simulink model "Consensus_Swarm"  (R2023b)
settings: Solver=ode3  StartTime=0.0  StopTime=inf  FixedStep=0.001  RelTol=1e-3
values from neighbouring files (symbols this model uses):
  g = 9.8    [Parameters.m]
  Ic = [2 0 0; 0 2 0; 0 0 4]    [Parameters.m]
  m = 1    [Parameters.m]
  M_RB = [eye(3), zeros(3); zeros(3), I]    [Parameters.m]
  SAVE_SPACE = 5    [Parameters.m]
  STEP_SIZE = 1    [Parameters.m]
libraries: simulink_extras x36, slpidlib x36, aerolibutil x12, vrlib x7
(part 1 of 6)
settings Model: Creator=angel  LastModifiedBy=angel

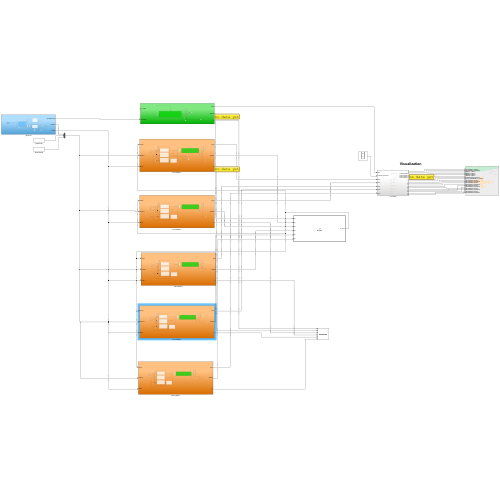
[thumbnail: Simulink's stored preview of the top-level diagram]
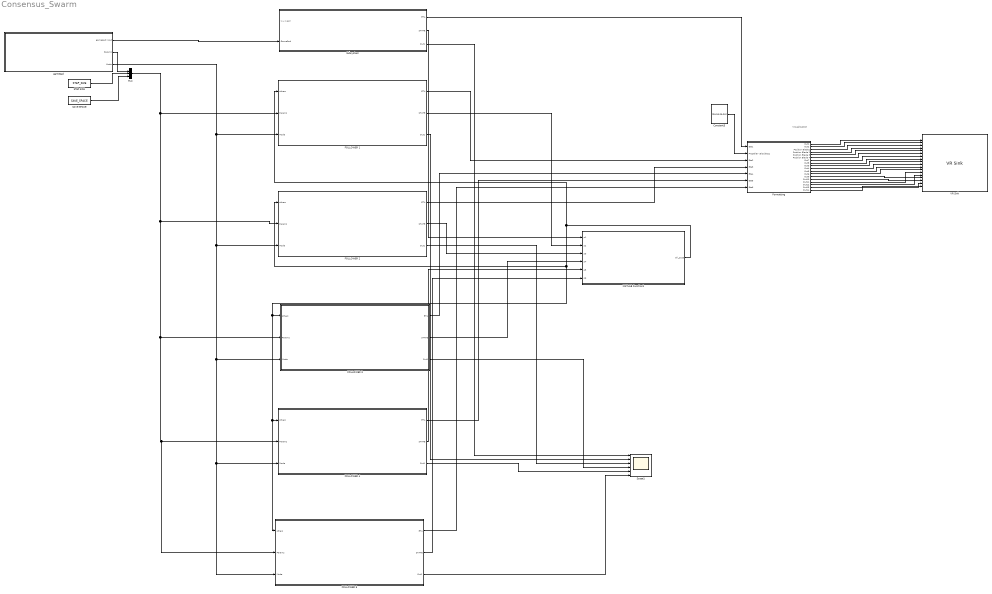
== system Consensus_Swarm ==
  note: Visualization
  Constant3 : Constant  Value=[20;20;20;20]  VectorParams1D=off
  FOLLOWER 1 : Subsystem
  FOLLOWER 2 : Subsystem
  FOLLOWER 3 : Subsystem
  FOLLOWER 4 : Subsystem
  FOLLOWER 5 : Subsystem
  Formatting : Subsystem
  MATLAB Function1 : MATLAB Function  TreatAsAtomicUnit=on
  Mux : Mux  Inputs=3
  SAVE SPACE : Constant  Value=SAVE_SPACE
  STEP SIZE : Constant  Value=STEP_SIZE
  Scope1 : Scope  NumInputPorts=6
  Subsystem : Subsystem
  VR Sink : vrlib/VR Sink  InstantiateOnLoad=on  SampleTime=12*0.005  ViewEnable=on  RemoteChange=off  RemoteView=off  FieldsWritten=QuadBody1.rotation.4.1.1.double#QuadBody1.translation.3.1.1.double#Blade1.rotation.4.1.1.double#Blade3.rotation.4.1.1.double#Blade2.rotation.4.1.1.double#Blade4.rotation.4.1.1.double#IsoNoRotation.position.3.1.1.double#OnQuadNoRotation.position.3.1.1.double#QuadBody2.rotation.4.1.1.double#QuadBody2.translation.3.1.1.double#QuadBody3.rotation.4.1.1.double#QuadBody3.translation.3.1.1.double#QuadBody5.rotation.4.1.1.double#QuadBody5.translation.3.1.1.double#QuadBody4.rotation.4.1.1.double#QuadBody4.translation.3.1.1.double#QuadBody6.rotation.4.1.1.double#QuadBody6.translation.3.1.1.double  WorldFileName=Quadcoptertwo_VR.wrl  AutoView=on  VideoDimensions=[]  AllowVariableSize=off  FigureProperties="{'Position', 'Name', 'Viewpoint', 'CameraBound', 'CameraDirection', 'CameraPosition', 'CameraUpVector', 'ZoomFactor', 'Antialiasing', 'Headlight', 'Lighting', 'NavPanel', 'Sound', 'StatusBar', 'Stereo3D', 'Stereo3DCameraOffset', 'Stereo3DHIT', 'ToolBar', 'Textures', 'Transparency', 'Triad', 'Wireframe', 'NavZones', 'NavMode', 'NavSpeed', 'CaptureFileFormat', 'CaptureFileName', 'Record2DCompressMethod', 'Record2DCompressQuality', 'Record2D', 'Record2DFileName', 'Record2DFPS'; [1.0000000000000000e+00   7.4199999999999932e+01   1.5360000000000000e+03   6.9080000000000007e+02], '', 'Isometric', 'on', [0.0000000000000000e+00   0.0000000000000000e+00  -1.0000000000000000e+00], [0.0000000000000000e+00   0.0000000000000000e+00   6.0000000000000000e+00], [0.0000000000000000e+00   1.0000000000000000e+00   0.0000000000000000e+00], [1.0000000000000000e+00], 'on', 'on', 'on', 'halfbar', 'on', 'on', 'off', [1.0000000149011612e-01], [0.0000000000000000e+00], 'on', 'on', 'on', 'none', 'off', 'off', 'fly', 'normal', 'tif', '%f_anim_%n.tif', 'auto', [7.5000000000000000e+01], 'off', '%f_anim_%n.avi', 'auto'}"
  gamepad : Subsystem
  wires:
  Constant3/1 -> Formatting/2(Propeller velocities1)
  gamepad/2(Params) -> Mux/1
  STEP SIZE/1 -> Mux/2
  Mux/1 -> FOLLOWER 2/2(Params), FOLLOWER 4/2(Params), FOLLOWER 5/2(Params), FOLLOWER 3/2(Params), FOLLOWER 1/2(Params)
  FOLLOWER 3/1(ETA) -> Formatting/5(Eta4)
  FOLLOWER 3/2(STATE) -> MATLAB Function1/4(p4)
  SAVE SPACE/1 -> Mux/3
  MATLAB Function1/1(all_pose) -> FOLLOWER 1/1(others), FOLLOWER 2/1(others), FOLLOWER 5/1(others), FOLLOWER 4/1(others), FOLLOWER 3/1(others)
  FOLLOWER 2/2(STATE) -> MATLAB Function1/3(p3)
  FOLLOWER 1/2(STATE) -> MATLAB Function1/2(p2)
  FOLLOWER 2/1(ETA) -> Formatting/4(Eta3)
  FOLLOWER 1/1(ETA) -> Formatting/3(Eta2)
  gamepad/1(gamepad input) -> Subsystem/2(GamePad)
  Subsystem/1(ETA) -> Formatting/1(Eta1)
  Subsystem/2(STATE) -> MATLAB Function1/1(p1)
  gamepad/3(Mode) -> FOLLOWER 5/3(Mode), FOLLOWER 4/3(Mode), FOLLOWER 3/3(Mode), FOLLOWER 2/3(Mode), FOLLOWER 1/3(Mode)
  Formatting/1(Out1) -> VR Sink/1
  Formatting/2(Out2) -> VR Sink/2
  Formatting/3(Position Blade1) -> VR Sink/3
  Formatting/4(Position Blade 2) -> VR Sink/4
  Formatting/5(Position Blade 3) -> VR Sink/5
  Formatting/6(Position Blade 4) -> VR Sink/6
  Formatting/7(Out7) -> VR Sink/7
  Formatting/8(Out8) -> VR Sink/8
  Formatting/9(Out3) -> VR Sink/9
  Formatting/10(Out4) -> VR Sink/10
  Formatting/11(Out5) -> VR Sink/11
  Formatting/12(Out6) -> VR Sink/12
  Formatting/13(Out9) -> VR Sink/15
  Formatting/14(Out10) -> VR Sink/16
  Formatting/15(Out11) -> VR Sink/13
  Formatting/16(Out12) -> VR Sink/14
  Formatting/17(Out13) -> VR Sink/17
  Formatting/18(Out14) -> VR Sink/18
  FOLLOWER 4/1(ETA) -> Formatting/6(Eta5)
  FOLLOWER 4/2(STATE) -> MATLAB Function1/5(p5)
  FOLLOWER 5/1(ETA) -> Formatting/7(Eta6)
  FOLLOWER 5/2(STATE) -> MATLAB Function1/6(p6)
  FOLLOWER 5/3(Out1) -> Scope1/6
  FOLLOWER 4/3(Out1) -> Scope1/5
  FOLLOWER 3/3(Out1) -> Scope1/4
  FOLLOWER 2/3(Out1) -> Scope1/3
  FOLLOWER 1/3(Out1) -> Scope1/2
  Subsystem/3(Out1) -> Scope1/1

== system Consensus_Swarm/FOLLOWER 1 ==
  others : Inport
  Params : Inport  Port=2
  Mode : Inport  Port=3
  Agent Model : Subsystem
  Demux : Demux
  Demux1 : Demux
  Demux3 : Demux  Outputs=6
  ID : Constant  Value=2
  MATLAB Function : MATLAB Function  TreatAsAtomicUnit=on
  MATLAB Function1 : MATLAB Function  TreatAsAtomicUnit=on
  MATLAB Function10 : MATLAB Function  TreatAsAtomicUnit=on
  MATLAB Function11 : MATLAB Function  TreatAsAtomicUnit=on
  Multiport Switch : MultiPortSwitch  SaturateOnIntegerOverflow=off  InputSameDT=off
  Mux4 : Mux
  Scope : Scope  NumInputPorts=2
  ETA : Outport
  STATE : Outport  Port=2
  Out1 : Outport  Port=3
  wires:
  MATLAB Function11/1(ref) -> Multiport Switch/2
  others/1 -> MATLAB Function10/3(others), MATLAB Function1/2(others), MATLAB Function/2(others), MATLAB Function11/2(others)
  Params/1 -> Demux/1
  ID/1 -> MATLAB Function10/1(id), MATLAB Function/1(id), MATLAB Function11/1(id), MATLAB Function1/1(id)
  Demux/1 -> MATLAB Function/4(d), MATLAB Function11/3(d)
  Demux/2 -> MATLAB Function11/4(phi)
  Demux/4 -> MATLAB Function10/4(safe_space)
  Demux/3 -> MATLAB Function11/5(base_speed), MATLAB Function1/3(base_speed), MATLAB Function/3(base_speed)
  Demux3/3 -> Mux4/3
  MATLAB Function1/1(ref) -> MATLAB Function10/2(ref)
  Mode/1 -> Multiport Switch/1
  MATLAB Function10/1(new_ref) -> Multiport Switch/4
  Agent Model/1(Eta) -> ETA/1, Demux3/1
  Multiport Switch/1 -> Agent Model/1((x,y,z,psi))
  Demux3/1 -> Mux4/1
  Demux3/2 -> Mux4/2
  Mux4/1 -> STATE/1
  Demux3/6 -> Out1/1, Mux4/4
  Demux1/4 -> Scope/1
  MATLAB Function/1(ref) -> Demux1/1, Multiport Switch/3
  MATLAB Function/2(angle) -> Scope/2

== system Consensus_Swarm/FOLLOWER 2 ==
  others : Inport
  Params : Inport  Port=2
  Mode : Inport  Port=3
  Agent Model : Subsystem
  Demux : Demux
  Demux3 : Demux  Outputs=6
  ID : Constant  Value=3
  MATLAB Function : MATLAB Function  TreatAsAtomicUnit=on
  MATLAB Function1 : MATLAB Function  TreatAsAtomicUnit=on
  MATLAB Function10 : MATLAB Function  TreatAsAtomicUnit=on
  MATLAB Function11 : MATLAB Function  TreatAsAtomicUnit=on
  Multiport Switch : MultiPortSwitch  SaturateOnIntegerOverflow=off  InputSameDT=off
  Mux4 : Mux
  ETA : Outport
  STATE : Outport  Port=2
  Out1 : Outport  Port=3
  wires:
  MATLAB Function11/1(ref) -> Multiport Switch/2
  others/1 -> MATLAB Function10/3(others), MATLAB Function1/2(others), MATLAB Function/2(others), MATLAB Function11/2(others)
  Params/1 -> Demux/1
  ID/1 -> MATLAB Function10/1(id), MATLAB Function/1(id), MATLAB Function11/1(id), MATLAB Function1/1(id)
  Demux/1 -> MATLAB Function/4(d), MATLAB Function11/3(d)
  Demux/2 -> MATLAB Function11/4(phi)
  Demux/4 -> MATLAB Function10/4(safe_space)
  Demux/3 -> MATLAB Function11/5(base_speed), MATLAB Function1/3(base_speed), MATLAB Function/3(base_speed)
  Demux3/3 -> Mux4/3
  MATLAB Function/1(ref) -> Multiport Switch/3
  MATLAB Function1/1(ref) -> MATLAB Function10/2(ref)
  Mode/1 -> Multiport Switch/1
  MATLAB Function10/1(new_ref) -> Multiport Switch/4
  Agent Model/1(Eta) -> ETA/1, Demux3/1
  Multiport Switch/1 -> Agent Model/1((x,y,z,psi))
  Demux3/1 -> Mux4/1
  Demux3/2 -> Mux4/2
  Mux4/1 -> STATE/1
  Demux3/6 -> Out1/1, Mux4/4

== system Consensus_Swarm/FOLLOWER 3 ==
  others : Inport
  Params : Inport  Port=2
  Mode : Inport  Port=3
  Agent Model : Subsystem
  Demux : Demux
  Demux3 : Demux  Outputs=6
  ID : Constant  Value=4
  MATLAB Function : MATLAB Function  TreatAsAtomicUnit=on
  MATLAB Function1 : MATLAB Function  TreatAsAtomicUnit=on
  MATLAB Function10 : MATLAB Function  TreatAsAtomicUnit=on
  MATLAB Function11 : MATLAB Function  TreatAsAtomicUnit=on
  Multiport Switch : MultiPortSwitch  SaturateOnIntegerOverflow=off  InputSameDT=off
  Mux4 : Mux
  ETA : Outport
  STATE : Outport  Port=2
  Out1 : Outport  Port=3
  wires:
  MATLAB Function11/1(ref) -> Multiport Switch/2
  others/1 -> MATLAB Function10/3(others), MATLAB Function1/2(others), MATLAB Function/2(others), MATLAB Function11/2(others)
  Params/1 -> Demux/1
  ID/1 -> MATLAB Function10/1(id), MATLAB Function/1(id), MATLAB Function11/1(id), MATLAB Function1/1(id)
  Demux/1 -> MATLAB Function/4(d), MATLAB Function11/3(d)
  Demux/2 -> MATLAB Function11/4(phi)
  Demux/4 -> MATLAB Function10/4(safe_space)
  Demux/3 -> MATLAB Function11/5(base_speed), MATLAB Function/3(base_speed), MATLAB Function1/3(base_speed)
  Demux3/3 -> Mux4/3
  MATLAB Function/1(ref) -> Multiport Switch/3
  MATLAB Function1/1(ref) -> MATLAB Function10/2(ref)
  Mode/1 -> Multiport Switch/1
  MATLAB Function10/1(new_ref) -> Multiport Switch/4
  Agent Model/1(Eta) -> ETA/1, Demux3/1
  Multiport Switch/1 -> Agent Model/1((x,y,z,psi))
  Demux3/1 -> Mux4/1
  Demux3/2 -> Mux4/2
  Mux4/1 -> STATE/1
  Demux3/6 -> Mux4/4, Out1/1

== system Consensus_Swarm/FOLLOWER 4 ==
  others : Inport
  Params : Inport  Port=2
  Mode : Inport  Port=3
  Agent Model : Subsystem
  Demux : Demux
  Demux3 : Demux  Outputs=6
  ID : Constant  Value=5
  MATLAB Function : MATLAB Function  TreatAsAtomicUnit=on
  MATLAB Function1 : MATLAB Function  TreatAsAtomicUnit=on
  MATLAB Function10 : MATLAB Function  TreatAsAtomicUnit=on
  MATLAB Function11 : MATLAB Function  TreatAsAtomicUnit=on
  Multiport Switch : MultiPortSwitch  SaturateOnIntegerOverflow=off  InputSameDT=off
  Mux4 : Mux
  ETA : Outport
  STATE : Outport  Port=2
  Out1 : Outport  Port=3
  wires:
  MATLAB Function11/1(ref) -> Multiport Switch/2
  others/1 -> MATLAB Function10/3(others), MATLAB Function1/2(others), MATLAB Function/2(others), MATLAB Function11/2(others)
  Params/1 -> Demux/1
  ID/1 -> MATLAB Function10/1(id), MATLAB Function/1(id), MATLAB Function11/1(id), MATLAB Function1/1(id)
  Demux/1 -> MATLAB Function/4(d), MATLAB Function11/3(d)
  Demux/2 -> MATLAB Function11/4(phi)
  Demux/4 -> MATLAB Function10/4(safe_space)
  Demux/3 -> MATLAB Function11/5(base_speed), MATLAB Function/3(base_speed), MATLAB Function1/3(base_speed)
  Demux3/3 -> Mux4/3
  MATLAB Function/1(ref) -> Multiport Switch/3
  MATLAB Function1/1(ref) -> MATLAB Function10/2(ref)
  Mode/1 -> Multiport Switch/1
  MATLAB Function10/1(new_ref) -> Multiport Switch/4
  Agent Model/1(Eta) -> ETA/1, Demux3/1
  Multiport Switch/1 -> Agent Model/1((x,y,z,psi))
  Demux3/1 -> Mux4/1
  Demux3/2 -> Mux4/2
  Mux4/1 -> STATE/1
  Demux3/6 -> Out1/1, Mux4/4

== system Consensus_Swarm/FOLLOWER 5 ==
  others : Inport
  Params : Inport  Port=2
  Mode : Inport  Port=3
  Agent Model : Subsystem
  Demux : Demux
  Demux3 : Demux  Outputs=6
  ID : Constant  Value=6
  MATLAB Function : MATLAB Function  TreatAsAtomicUnit=on
  MATLAB Function1 : MATLAB Function  TreatAsAtomicUnit=on
  MATLAB Function10 : MATLAB Function  TreatAsAtomicUnit=on
  MATLAB Function11 : MATLAB Function  TreatAsAtomicUnit=on
  Multiport Switch : MultiPortSwitch  SaturateOnIntegerOverflow=off  InputSameDT=off
  Mux4 : Mux
  ETA : Outport
  STATE : Outport  Port=2
  Out1 : Outport  Port=3
  wires:
  MATLAB Function11/1(ref) -> Multiport Switch/2
  others/1 -> MATLAB Function10/3(others), MATLAB Function1/2(others), MATLAB Function/2(others), MATLAB Function11/2(others)
  Params/1 -> Demux/1
  ID/1 -> MATLAB Function10/1(id), MATLAB Function/1(id), MATLAB Function11/1(id), MATLAB Function1/1(id)
  Demux/1 -> MATLAB Function/4(d), MATLAB Function11/3(d)
  Demux/2 -> MATLAB Function11/4(phi)
  Demux/4 -> MATLAB Function10/4(safe_space)
  Demux/3 -> MATLAB Function11/5(base_speed), MATLAB Function/3(base_speed), MATLAB Function1/3(base_speed)
  Demux3/3 -> Mux4/3
  MATLAB Function/1(ref) -> Multiport Switch/3
  MATLAB Function1/1(ref) -> MATLAB Function10/2(ref)
  Mode/1 -> Multiport Switch/1
  MATLAB Function10/1(new_ref) -> Multiport Switch/4
  Agent Model/1(Eta) -> ETA/1, Demux3/1
  Multiport Switch/1 -> Agent Model/1((x,y,z,psi))
  Demux3/1 -> Mux4/1
  Demux3/2 -> Mux4/2
  Mux4/1 -> STATE/1
  Demux3/6 -> Out1/1, Mux4/4

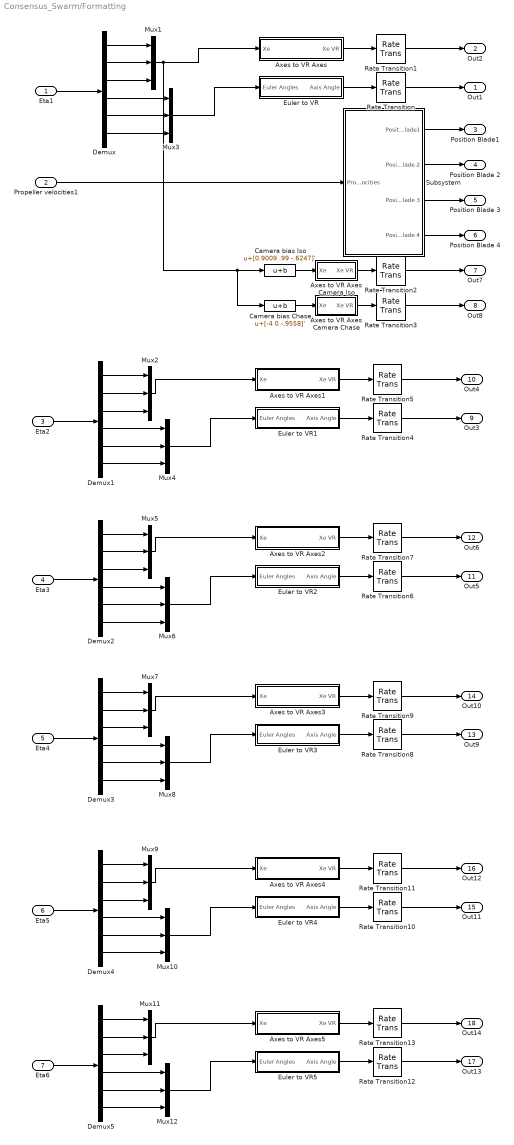
== system Consensus_Swarm/Formatting ==
  Eta1 : Inport
  Propeller velocities1 : Inport  Port=2
  Eta2 : Inport  Port=3
  Eta3 : Inport  Port=4
  Eta4 : Inport  Port=5
  Eta5 : Inport  Port=6
  Eta6 : Inport  Port=7
  Axes to VR Axes : Subsystem
  Axes to VR Axes Camera Chase : Subsystem
  Axes to VR Axes Camera Iso : Subsystem
  Axes to VR Axes1 : Subsystem
  Axes to VR Axes2 : Subsystem
  Axes to VR Axes3 : Subsystem
  Axes to VR Axes4 : Subsystem
  Axes to VR Axes5 : Subsystem
  Camera bias Chase : Bias  Bias=[-4 0 -.9558]'  SaturateOnIntegerOverflow=off
  Camera bias Iso : Bias  Bias=[0.9009 .99 -.6247]'  SaturateOnIntegerOverflow=off
  Demux{,1..5} (6 alike) : Demux  Outputs=6
  Euler to VR : Subsystem
  Euler to VR1 : Subsystem
  Euler to VR2 : Subsystem
  Euler to VR3 : Subsystem
  Euler to VR4 : Subsystem
  Euler to VR5 : Subsystem
  Mux{1..12} (12 alike) : Mux  Inputs=3
  Rate Transition{,1..13} (14 alike) : RateTransition
  Subsystem : Subsystem
  Out1 : Outport
  Out2 : Outport  Port=2
  Position Blade1 : Outport  Port=3
  Position Blade 2 : Outport  Port=4
  Position Blade 3 : Outport  Port=5
  Position Blade 4 : Outport  Port=6
  Out7 : Outport  Port=7
  Out8 : Outport  Port=8
  Out3 : Outport  Port=9
  Out4 : Outport  Port=10
  Out5 : Outport  Port=11
  Out6 : Outport  Port=12
  Out9 : Outport  Port=13
  Out10 : Outport  Port=14
  Out11 : Outport  Port=15
  Out12 : Outport  Port=16
  Out13 : Outport  Port=17
  Out14 : Outport  Port=18
  wires:
  Rate Transition2/1 -> Out7/1
  Propeller velocities1/1 -> Subsystem/1(Propeller velocities)
  Subsystem/3(Position Blade 3) -> Position Blade 3/1
  Subsystem/1(Position Blade1) -> Position Blade1/1
  Mux3/1 -> Euler to VR/1(Euler Angles)
  Camera bias Chase/1 -> Axes to VR Axes Camera Chase/1(Xe)
  Axes to VR Axes Camera Chase/1(Xe VR) -> Rate Transition3/1
  Subsystem/2(Position Blade 2) -> Position Blade 2/1
  Axes to VR Axes Camera Iso/1(Xe VR) -> Rate Transition2/1
  Euler to VR/1(Axis Angle) -> Rate Transition/1
  Axes to VR Axes/1(Xe VR) -> Rate Transition1/1
  Rate Transition1/1 -> Out2/1
  Camera bias Iso/1 -> Axes to VR Axes Camera Iso/1(Xe)
  Mux1/1 -> Camera bias Chase/1, Camera bias Iso/1, Axes to VR Axes/1(Xe)
  Rate Transition3/1 -> Out8/1
  Rate Transition/1 -> Out1/1
  Subsystem/4(Position Blade 4) -> Position Blade 4/1
  Demux/2 -> Mux1/2
  Demux/5 -> Mux3/2
  Demux/3 -> Mux1/3
  Eta1/1 -> Demux/1
  Demux/1 -> Mux1/1
  Demux/4 -> Mux3/1
  Demux/6 -> Mux3/3
  Demux1/3 -> Mux2/3
  Demux1/1 -> Mux2/1
  Euler to VR1/1(Axis Angle) -> Rate Transition4/1
  Mux2/1 -> Axes to VR Axes1/1(Xe)
  Eta2/1 -> Demux1/1
  Axes to VR Axes1/1(Xe VR) -> Rate Transition5/1
  Rate Transition5/1 -> Out4/1
  Mux4/1 -> Euler to VR1/1(Euler Angles)
  Demux1/4 -> Mux4/1
  Demux1/2 -> Mux2/2
  Rate Transition4/1 -> Out3/1
  Demux1/5 -> Mux4/2
  Demux1/6 -> Mux4/3
  Mux6/1 -> Euler to VR2/1(Euler Angles)
  Demux2/6 -> Mux6/3
  Demux2/5 -> Mux6/2
  Rate Transition6/1 -> Out5/1
  Demux2/2 -> Mux5/2
  Demux2/4 -> Mux6/1
  Eta3/1 -> Demux2/1
  Euler to VR2/1(Axis Angle) -> Rate Transition6/1
  Axes to VR Axes2/1(Xe VR) -> Rate Transition7/1
  Demux2/1 -> Mux5/1
  Rate Transition7/1 -> Out6/1
  Demux2/3 -> Mux5/3
  Mux5/1 -> Axes to VR Axes2/1(Xe)
  Demux3/3 -> Mux7/3
  Mux7/1 -> Axes to VR Axes3/1(Xe)
  Rate Transition9/1 -> Out10/1
  Demux3/6 -> Mux8/3
  Eta4/1 -> Demux3/1
  Euler to VR3/1(Axis Angle) -> Rate Transition8/1
  Demux3/2 -> Mux7/2
  Demux3/4 -> Mux8/1
  Demux3/1 -> Mux7/1
  Rate Transition8/1 -> Out9/1
  Axes to VR Axes3/1(Xe VR) -> Rate Transition9/1
  Demux3/5 -> Mux8/2
  Mux8/1 -> Euler to VR3/1(Euler Angles)
  Demux4/5 -> Mux10/2
  Rate Transition10/1 -> Out11/1
  Mux10/1 -> Euler to VR4/1(Euler Angles)
  Demux4/2 -> Mux9/2
  Rate Transition11/1 -> Out12/1
  Demux4/3 -> Mux9/3
  Euler to VR4/1(Axis Angle) -> Rate Transition10/1
  Eta5/1 -> Demux4/1
  Demux4/6 -> Mux10/3
  Demux4/4 -> Mux10/1
  Mux9/1 -> Axes to VR Axes4/1(Xe)
  Demux4/1 -> Mux9/1
  Axes to VR Axes4/1(Xe VR) -> Rate Transition11/1
  Demux5/5 -> Mux12/2
  Rate Transition12/1 -> Out13/1
  Mux12/1 -> Euler to VR5/1(Euler Angles)
  Demux5/2 -> Mux11/2
  Rate Transition13/1 -> Out14/1
  Demux5/3 -> Mux11/3
  Euler to VR5/1(Axis Angle) -> Rate Transition12/1
  Eta6/1 -> Demux5/1
  Demux5/6 -> Mux12/3
  Demux5/4 -> Mux12/1
  Mux11/1 -> Axes to VR Axes5/1(Xe)
  Demux5/1 -> Mux11/1
  Axes to VR Axes5/1(Xe VR) -> Rate Transition13/1

== system Consensus_Swarm/Subsystem ==
  (x,y,z,psi) : Inport
  GamePad : Inport  Port=2
  Demux3 : Demux  Outputs=6
  LIDER : Subsystem
      settings: PortSchema="{\"entries\":[{\"content\":{\"sides\":[{\"content\":{\"connectorIds\":[\"In1\"]},\"type\":\"ConnectorPlacement.EquallySpacedRectSide\",\"uuid\":\"c8d85519-df1b-4853-9438-4e257db698fb\"},{\"content\":{\"connectorIds\":[\"Out1\"],\"side\":\"RIGHT\"},\"type\":\"ConnectorPlacement.EquallySpacedRectSide\",\"uuid\":\"bb73f18c-f7b2-42f7-b6a6-cc8929734169\"},{\"content\":{\"connectorIds\":[\"In2\"],\"side\":\"TOP\"},\"type\":\"ConnectorPlacement.EquallySpacedRectSide\",\"uuid\":\"c63c7747-484c-49ed-9b90-ed1a1a5ff702\"}]},\"type\":\"ConnectorPlacement.EquallySpacedConnector\",\"uuid\":\"1f845c39-dafc-4c76-a00d-fc51587114d9\"}],\"packageUris\":[\"http://schema.mathworks.com/mf0/Connector/R2020b\"],\"version\":\"1.0\"}"
  Mux4 : Mux
  ETA : Outport
  STATE : Outport  Port=2
  Out1 : Outport  Port=3
  wires:
  LIDER/1(Eta) -> ETA/1, Demux3/1
  Demux3/3 -> Mux4/3
  Mux4/1 -> STATE/1
  Demux3/2 -> Mux4/2
  Demux3/1 -> Mux4/1
  GamePad/1 -> LIDER/2(GamePad)
  (x,y,z,psi)/1 -> LIDER/1((x,y,z,psi))
  Demux3/6 -> Out1/1, Mux4/4

== system Consensus_Swarm/gamepad ==
  Formatting : Subsystem
  Gamepad : vrlib/Joystick Input  joyid=1  adjustports=on  forcefeed=off
  MATLAB Function : MATLAB Function  TreatAsAtomicUnit=on
  MATLAB Function7 : MATLAB Function  TreatAsAtomicUnit=on
  Mux : Mux  Inputs=2
  Saturation1 : Saturate  UpperLimit=10  LowerLimit=-10
  Saturation2 : Saturate  UpperLimit=pi  LowerLimit=-pi
  Saturation3 : Saturate  UpperLimit=10  LowerLimit=0
  Scope : Scope  NumInputPorts=2
  Scope1 : Scope
  Scope2 : Scope
  Unit Delay : UnitDelay  SampleTime=-1  HasFrameUpgradeWarning=on
  Unit Delay1 : UnitDelay  SampleTime=-1  HasFrameUpgradeWarning=on
  Unit Delay2 : UnitDelay  InitialCondition=3  SampleTime=-1  HasFrameUpgradeWarning=on
  Zero-Order Hold : ZeroOrderHold  SampleTime=-1
  Zero-Order Hold1 : ZeroOrderHold  SampleTime=-1
  gamepad input : Outport
  Params : Outport  Port=2
  Mode : Outport  Port=3
  wires:
  Gamepad/1 -> Scope1/1, Formatting/1(Axes)
  Zero-Order Hold1/1 -> Saturation1/1
  Gamepad/2 -> Scope2/1, Formatting/2(Buttons)
  Formatting/1("Altitude, Roll, Pitch, Yaw") -> gamepad input/1
  Formatting/6(Scale Factor) -> Zero-Order Hold1/1
  Unit Delay1/1 -> MATLAB Function7/4(phi)
  Formatting/7(Rotation Factor) -> Zero-Order Hold/1
  Unit Delay/1 -> MATLAB Function7/3(d)
  Zero-Order Hold/1 -> Saturation2/1
  MATLAB Function7/1(d_new) -> Unit Delay/1, Scope/2, Saturation3/1
  Saturation1/1 -> MATLAB Function7/1(scale_factor)
  Saturation2/1 -> MATLAB Function7/2(angle_factor)
  Mux/1 -> Params/1
  MATLAB Function/1(new_mode) -> Mode/1, Unit Delay2/1
  Unit Delay2/1 -> MATLAB Function/4(mode)
  Formatting/4(Square) -> MATLAB Function/3(square)
  Formatting/3(Circle) -> MATLAB Function/2(circle)
  Formatting/2(Cross) -> MATLAB Function/1(x)
  Saturation3/1 -> Mux/1
  MATLAB Function7/2(phi_new) -> Unit Delay1/1, Mux/2, Scope/1

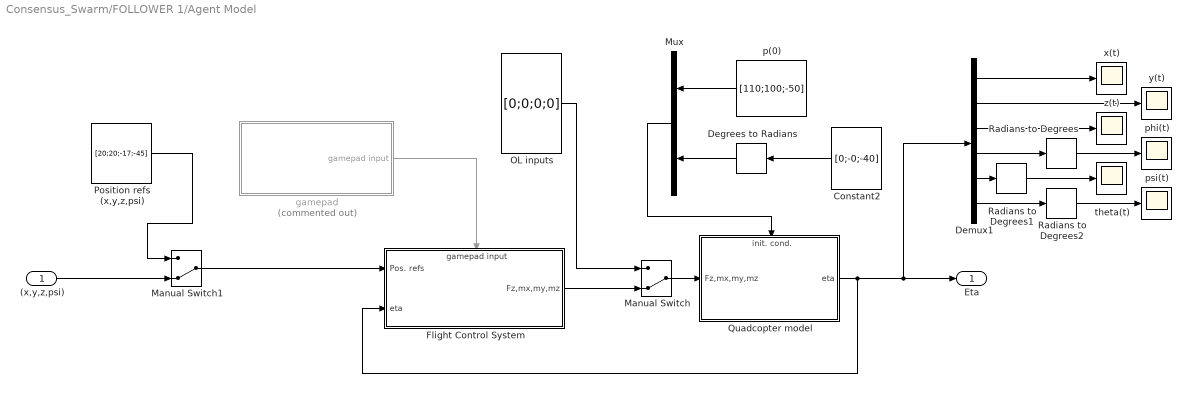
== system Consensus_Swarm/FOLLOWER 1/Agent Model ==
  (x,y,z,psi) : Inport
  Constant2 : Constant  Value=[0;-0;-40]  VectorParams1D=off
  Degrees to Radians : simulink_extras/Transformations/Degrees to Radians
  Demux1 : Demux  Outputs=6
  Flight Control System : Subsystem
      settings: PortSchema="{\"entries\":[{\"content\":{\"sides\":[{\"content\":{\"connectorIds\":[\"In1\",\"In2\"]},\"type\":\"ConnectorPlacement.EquallySpacedRectSide\",\"uuid\":\"8ffec179-99fb-4b4c-a09d-a73fa0154dea\"},{\"content\":{\"connectorIds\":[\"Out1\"],\"side\":\"RIGHT\"},\"type\":\"ConnectorPlacement.EquallySpacedRectSide\",\"uuid\":\"b9ff487d-1da1-449a-81c9-f1838b0d3727\"},{\"content\":{\"connectorIds\":[\"In3\"],\"side\":\"TOP\"},\"type\":\"ConnectorPlacement.EquallySpacedRectSide\",\"uuid\":\"1948ac9a-8b1f-4a62-833b-18e2b106d39d\"}]},\"type\":\"ConnectorPlacement.EquallySpacedConnector\",\"uuid\":\"fea635f7-9753-4696-bad7-e2485c1b5acc\"}],\"packageUris\":[\"http://schema.mathworks.com/mf0/Connector/R2020b\"],\"version\":\"1.0\"}"
  Manual Switch : ManualSwitch  CurrentSetting=0
  Manual Switch1 : ManualSwitch  CurrentSetting=0
  Mux : Mux  Inputs=2
  OL inputs : Constant  Value=[0;0;0;0]  VectorParams1D=off
  Position refs (x,y,z,psi) : Constant  Value=[20;20;-17;-45]  VectorParams1D=off
  Quadcopter model : Subsystem
      settings: PortSchema="{\"entries\":[{\"content\":{\"sides\":[{\"content\":{\"connectorIds\":[\"In1\"]},\"type\":\"ConnectorPlacement.EquallySpacedRectSide\",\"uuid\":\"c5c2dfb8-9ff8-4aa4-96a6-7fa0d886c51f\"},{\"content\":{\"connectorIds\":[\"Out1\"],\"side\":\"RIGHT\"},\"type\":\"ConnectorPlacement.EquallySpacedRectSide\",\"uuid\":\"2d7c7d5c-4ac5-4ebd-b09f-6a78733e851d\"},{\"content\":{\"connectorIds\":[\"In2\"],\"side\":\"TOP\"},\"type\":\"ConnectorPlacement.EquallySpacedRectSide\",\"uuid\":\"cf3a786d-06ed-46d4-985b-5c210afb13ec\"}]},\"type\":\"ConnectorPlacement.EquallySpacedConnector\",\"uuid\":\"cd57f0e6-7b9c-4392-8478-6e8af8e2560e\"}],\"packageUris\":[\"http://schema.mathworks.com/mf0/Connector/R2020b\"],\"version\":\"1.0\"}"
  Radians to Degrees : simulink_extras/Transformations/Radians to Degrees
  Radians to Degrees1 : simulink_extras/Transformations/Radians to Degrees
  Radians to Degrees2 : simulink_extras/Transformations/Radians to Degrees
  gamepad : Subsystem  Commented=on
  p(0) : Constant  Value=[110;100;-50]  VectorParams1D=off
  phi(t) : Scope
  psi(t) : Scope
  theta(t) : Scope
  x(t) : Scope
  y(t) : Scope
  z(t) : Scope
  Eta : Outport
  wires:
  Radians to Degrees2/1 -> psi(t)/1
  Quadcopter model/1(eta) -> Eta/1, Demux1/1, Flight Control System/2(eta)
  OL inputs/1 -> Manual Switch/1
  Demux1/2 -> y(t)/1
  Constant2/1 -> Degrees to Radians/1
  gamepad/1(gamepad input) -> Flight Control System/3(gamepad input)
  p(0)/1 -> Mux/1
  Degrees to Radians/1 -> Mux/2
  Demux1/1 -> x(t)/1
  Radians to Degrees/1 -> phi(t)/1
  Demux1/4 -> Radians to Degrees/1
  Manual Switch1/1 -> Flight Control System/1(Pos. refs)
  Radians to Degrees1/1 -> theta(t)/1
  Demux1/3 -> z(t)/1
  Demux1/6 -> Radians to Degrees2/1
  Manual Switch/1 -> Quadcopter model/1(Fz,mx,my,mz)
  Demux1/5 -> Radians to Degrees1/1
  Position refs (x,y,z,psi)/1 -> Manual Switch1/1
  Flight Control System/1(Fz,mx,my,mz) -> Manual Switch/2
  Mux/1 -> Quadcopter model/2(init. cond.)
  (x,y,z,psi)/1 -> Manual Switch1/2

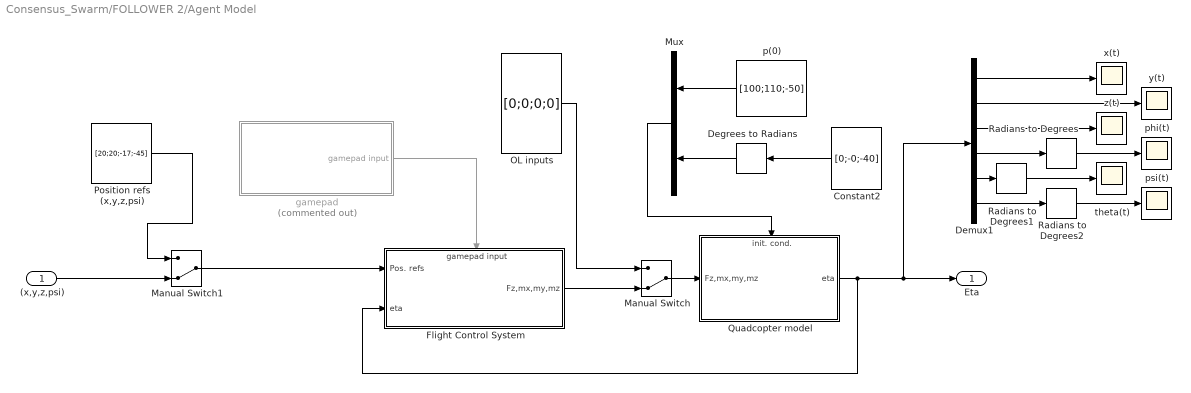
== system Consensus_Swarm/FOLLOWER 2/Agent Model ==
  (x,y,z,psi) : Inport
  Constant2 : Constant  Value=[0;-0;-40]  VectorParams1D=off
  Degrees to Radians : simulink_extras/Transformations/Degrees to Radians
  Demux1 : Demux  Outputs=6
  Flight Control System : Subsystem
      settings: PortSchema="{\"entries\":[{\"content\":{\"sides\":[{\"content\":{\"connectorIds\":[\"In1\",\"In2\"]},\"type\":\"ConnectorPlacement.EquallySpacedRectSide\",\"uuid\":\"8ffec179-99fb-4b4c-a09d-a73fa0154dea\"},{\"content\":{\"connectorIds\":[\"Out1\"],\"side\":\"RIGHT\"},\"type\":\"ConnectorPlacement.EquallySpacedRectSide\",\"uuid\":\"b9ff487d-1da1-449a-81c9-f1838b0d3727\"},{\"content\":{\"connectorIds\":[\"In3\"],\"side\":\"TOP\"},\"type\":\"ConnectorPlacement.EquallySpacedRectSide\",\"uuid\":\"1948ac9a-8b1f-4a62-833b-18e2b106d39d\"}]},\"type\":\"ConnectorPlacement.EquallySpacedConnector\",\"uuid\":\"fea635f7-9753-4696-bad7-e2485c1b5acc\"}],\"packageUris\":[\"http://schema.mathworks.com/mf0/Connector/R2020b\"],\"version\":\"1.0\"}"
  Manual Switch : ManualSwitch  CurrentSetting=0
  Manual Switch1 : ManualSwitch  CurrentSetting=0
  Mux : Mux  Inputs=2
  OL inputs : Constant  Value=[0;0;0;0]  VectorParams1D=off
  Position refs (x,y,z,psi) : Constant  Value=[20;20;-17;-45]  VectorParams1D=off
  Quadcopter model : Subsystem
      settings: PortSchema="{\"entries\":[{\"content\":{\"sides\":[{\"content\":{\"connectorIds\":[\"In1\"]},\"type\":\"ConnectorPlacement.EquallySpacedRectSide\",\"uuid\":\"c5c2dfb8-9ff8-4aa4-96a6-7fa0d886c51f\"},{\"content\":{\"connectorIds\":[\"Out1\"],\"side\":\"RIGHT\"},\"type\":\"ConnectorPlacement.EquallySpacedRectSide\",\"uuid\":\"2d7c7d5c-4ac5-4ebd-b09f-6a78733e851d\"},{\"content\":{\"connectorIds\":[\"In2\"],\"side\":\"TOP\"},\"type\":\"ConnectorPlacement.EquallySpacedRectSide\",\"uuid\":\"cf3a786d-06ed-46d4-985b-5c210afb13ec\"}]},\"type\":\"ConnectorPlacement.EquallySpacedConnector\",\"uuid\":\"cd57f0e6-7b9c-4392-8478-6e8af8e2560e\"}],\"packageUris\":[\"http://schema.mathworks.com/mf0/Connector/R2020b\"],\"version\":\"1.0\"}"
  Radians to Degrees : simulink_extras/Transformations/Radians to Degrees
  Radians to Degrees1 : simulink_extras/Transformations/Radians to Degrees
  Radians to Degrees2 : simulink_extras/Transformations/Radians to Degrees
  gamepad : Subsystem  Commented=on
  p(0) : Constant  Value=[100;110;-50]  VectorParams1D=off
  phi(t) : Scope
  psi(t) : Scope
  theta(t) : Scope
  x(t) : Scope
  y(t) : Scope
  z(t) : Scope
  Eta : Outport
  wires:
  Radians to Degrees2/1 -> psi(t)/1
  Quadcopter model/1(eta) -> Eta/1, Demux1/1, Flight Control System/2(eta)
  OL inputs/1 -> Manual Switch/1
  Demux1/2 -> y(t)/1
  Constant2/1 -> Degrees to Radians/1
  gamepad/1(gamepad input) -> Flight Control System/3(gamepad input)
  p(0)/1 -> Mux/1
  Degrees to Radians/1 -> Mux/2
  Demux1/1 -> x(t)/1
  Radians to Degrees/1 -> phi(t)/1
  Demux1/4 -> Radians to Degrees/1
  Manual Switch1/1 -> Flight Control System/1(Pos. refs)
  Radians to Degrees1/1 -> theta(t)/1
  Demux1/3 -> z(t)/1
  Demux1/6 -> Radians to Degrees2/1
  Manual Switch/1 -> Quadcopter model/1(Fz,mx,my,mz)
  Demux1/5 -> Radians to Degrees1/1
  Position refs (x,y,z,psi)/1 -> Manual Switch1/1
  Flight Control System/1(Fz,mx,my,mz) -> Manual Switch/2
  Mux/1 -> Quadcopter model/2(init. cond.)
  (x,y,z,psi)/1 -> Manual Switch1/2

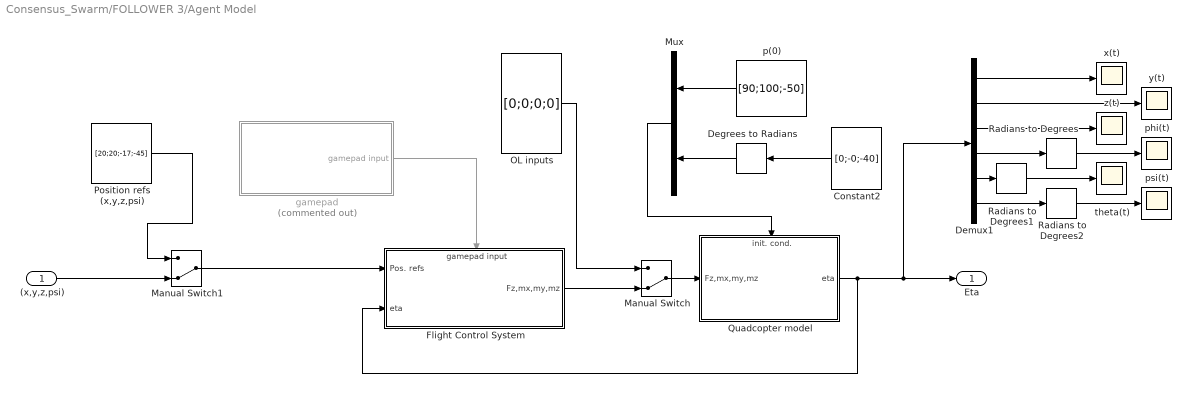
== system Consensus_Swarm/FOLLOWER 3/Agent Model ==
  (x,y,z,psi) : Inport
  Constant2 : Constant  Value=[0;-0;-40]  VectorParams1D=off
  Degrees to Radians : simulink_extras/Transformations/Degrees to Radians
  Demux1 : Demux  Outputs=6
  Flight Control System : Subsystem
      settings: PortSchema="{\"entries\":[{\"content\":{\"sides\":[{\"content\":{\"connectorIds\":[\"In1\",\"In2\"]},\"type\":\"ConnectorPlacement.EquallySpacedRectSide\",\"uuid\":\"8ffec179-99fb-4b4c-a09d-a73fa0154dea\"},{\"content\":{\"connectorIds\":[\"Out1\"],\"side\":\"RIGHT\"},\"type\":\"ConnectorPlacement.EquallySpacedRectSide\",\"uuid\":\"b9ff487d-1da1-449a-81c9-f1838b0d3727\"},{\"content\":{\"connectorIds\":[\"In3\"],\"side\":\"TOP\"},\"type\":\"ConnectorPlacement.EquallySpacedRectSide\",\"uuid\":\"1948ac9a-8b1f-4a62-833b-18e2b106d39d\"}]},\"type\":\"ConnectorPlacement.EquallySpacedConnector\",\"uuid\":\"fea635f7-9753-4696-bad7-e2485c1b5acc\"}],\"packageUris\":[\"http://schema.mathworks.com/mf0/Connector/R2020b\"],\"version\":\"1.0\"}"
  Manual Switch : ManualSwitch  CurrentSetting=0
  Manual Switch1 : ManualSwitch  CurrentSetting=0
  Mux : Mux  Inputs=2
  OL inputs : Constant  Value=[0;0;0;0]  VectorParams1D=off
  Position refs (x,y,z,psi) : Constant  Value=[20;20;-17;-45]  VectorParams1D=off
  Quadcopter model : Subsystem
      settings: PortSchema="{\"entries\":[{\"content\":{\"sides\":[{\"content\":{\"connectorIds\":[\"In1\"]},\"type\":\"ConnectorPlacement.EquallySpacedRectSide\",\"uuid\":\"c5c2dfb8-9ff8-4aa4-96a6-7fa0d886c51f\"},{\"content\":{\"connectorIds\":[\"Out1\"],\"side\":\"RIGHT\"},\"type\":\"ConnectorPlacement.EquallySpacedRectSide\",\"uuid\":\"2d7c7d5c-4ac5-4ebd-b09f-6a78733e851d\"},{\"content\":{\"connectorIds\":[\"In2\"],\"side\":\"TOP\"},\"type\":\"ConnectorPlacement.EquallySpacedRectSide\",\"uuid\":\"cf3a786d-06ed-46d4-985b-5c210afb13ec\"}]},\"type\":\"ConnectorPlacement.EquallySpacedConnector\",\"uuid\":\"cd57f0e6-7b9c-4392-8478-6e8af8e2560e\"}],\"packageUris\":[\"http://schema.mathworks.com/mf0/Connector/R2020b\"],\"version\":\"1.0\"}"
  Radians to Degrees : simulink_extras/Transformations/Radians to Degrees
  Radians to Degrees1 : simulink_extras/Transformations/Radians to Degrees
  Radians to Degrees2 : simulink_extras/Transformations/Radians to Degrees
  gamepad : Subsystem  Commented=on
  p(0) : Constant  Value=[90;100;-50]  VectorParams1D=off
  phi(t) : Scope
  psi(t) : Scope
  theta(t) : Scope
  x(t) : Scope
  y(t) : Scope
  z(t) : Scope
  Eta : Outport
  wires:
  Radians to Degrees2/1 -> psi(t)/1
  Quadcopter model/1(eta) -> Eta/1, Demux1/1, Flight Control System/2(eta)
  OL inputs/1 -> Manual Switch/1
  Demux1/2 -> y(t)/1
  Constant2/1 -> Degrees to Radians/1
  gamepad/1(gamepad input) -> Flight Control System/3(gamepad input)
  p(0)/1 -> Mux/1
  Degrees to Radians/1 -> Mux/2
  Demux1/1 -> x(t)/1
  Radians to Degrees/1 -> phi(t)/1
  Demux1/4 -> Radians to Degrees/1
  Manual Switch1/1 -> Flight Control System/1(Pos. refs)
  Radians to Degrees1/1 -> theta(t)/1
  Demux1/3 -> z(t)/1
  Demux1/6 -> Radians to Degrees2/1
  Manual Switch/1 -> Quadcopter model/1(Fz,mx,my,mz)
  Demux1/5 -> Radians to Degrees1/1
  Position refs (x,y,z,psi)/1 -> Manual Switch1/1
  Flight Control System/1(Fz,mx,my,mz) -> Manual Switch/2
  Mux/1 -> Quadcopter model/2(init. cond.)
  (x,y,z,psi)/1 -> Manual Switch1/2

== system Consensus_Swarm/FOLLOWER 4/Agent Model ==
  (x,y,z,psi) : Inport
  Constant2 : Constant  Value=[0;-0;-40]  VectorParams1D=off
  Degrees to Radians : simulink_extras/Transformations/Degrees to Radians
  Demux1 : Demux  Outputs=6
  Flight Control System : Subsystem
      settings: PortSchema="{\"entries\":[{\"content\":{\"sides\":[{\"content\":{\"connectorIds\":[\"In1\",\"In2\"]},\"type\":\"ConnectorPlacement.EquallySpacedRectSide\",\"uuid\":\"8ffec179-99fb-4b4c-a09d-a73fa0154dea\"},{\"content\":{\"connectorIds\":[\"Out1\"],\"side\":\"RIGHT\"},\"type\":\"ConnectorPlacement.EquallySpacedRectSide\",\"uuid\":\"b9ff487d-1da1-449a-81c9-f1838b0d3727\"},{\"content\":{\"connectorIds\":[\"In3\"],\"side\":\"TOP\"},\"type\":\"ConnectorPlacement.EquallySpacedRectSide\",\"uuid\":\"1948ac9a-8b1f-4a62-833b-18e2b106d39d\"}]},\"type\":\"ConnectorPlacement.EquallySpacedConnector\",\"uuid\":\"fea635f7-9753-4696-bad7-e2485c1b5acc\"}],\"packageUris\":[\"http://schema.mathworks.com/mf0/Connector/R2020b\"],\"version\":\"1.0\"}"
  Manual Switch : ManualSwitch  CurrentSetting=0
  Manual Switch1 : ManualSwitch  CurrentSetting=0
  Mux : Mux  Inputs=2
  OL inputs : Constant  Value=[0;0;0;0]  VectorParams1D=off
  Position refs (x,y,z,psi) : Constant  Value=[20;20;-17;-45]  VectorParams1D=off
  Quadcopter model : Subsystem
      settings: PortSchema="{\"entries\":[{\"content\":{\"sides\":[{\"content\":{\"connectorIds\":[\"In1\"]},\"type\":\"ConnectorPlacement.EquallySpacedRectSide\",\"uuid\":\"c5c2dfb8-9ff8-4aa4-96a6-7fa0d886c51f\"},{\"content\":{\"connectorIds\":[\"Out1\"],\"side\":\"RIGHT\"},\"type\":\"ConnectorPlacement.EquallySpacedRectSide\",\"uuid\":\"2d7c7d5c-4ac5-4ebd-b09f-6a78733e851d\"},{\"content\":{\"connectorIds\":[\"In2\"],\"side\":\"TOP\"},\"type\":\"ConnectorPlacement.EquallySpacedRectSide\",\"uuid\":\"cf3a786d-06ed-46d4-985b-5c210afb13ec\"}]},\"type\":\"ConnectorPlacement.EquallySpacedConnector\",\"uuid\":\"cd57f0e6-7b9c-4392-8478-6e8af8e2560e\"}],\"packageUris\":[\"http://schema.mathworks.com/mf0/Connector/R2020b\"],\"version\":\"1.0\"}"
  Radians to Degrees : simulink_extras/Transformations/Radians to Degrees
  Radians to Degrees1 : simulink_extras/Transformations/Radians to Degrees
  Radians to Degrees2 : simulink_extras/Transformations/Radians to Degrees
  gamepad : Subsystem  Commented=on
  p(0) : Constant  Value=[100;90;-50]  VectorParams1D=off
  phi(t) : Scope
  psi(t) : Scope
  theta(t) : Scope
  x(t) : Scope
  y(t) : Scope
  z(t) : Scope
  Eta : Outport
  wires:
  Radians to Degrees2/1 -> psi(t)/1
  Quadcopter model/1(eta) -> Eta/1, Demux1/1, Flight Control System/2(eta)
  OL inputs/1 -> Manual Switch/1
  Demux1/2 -> y(t)/1
  Constant2/1 -> Degrees to Radians/1
  gamepad/1(gamepad input) -> Flight Control System/3(gamepad input)
  p(0)/1 -> Mux/1
  Degrees to Radians/1 -> Mux/2
  Demux1/1 -> x(t)/1
  Radians to Degrees/1 -> phi(t)/1
  Demux1/4 -> Radians to Degrees/1
  Manual Switch1/1 -> Flight Control System/1(Pos. refs)
  Radians to Degrees1/1 -> theta(t)/1
  Demux1/3 -> z(t)/1
  Demux1/6 -> Radians to Degrees2/1
  Manual Switch/1 -> Quadcopter model/1(Fz,mx,my,mz)
  Demux1/5 -> Radians to Degrees1/1
  Position refs (x,y,z,psi)/1 -> Manual Switch1/1
  Flight Control System/1(Fz,mx,my,mz) -> Manual Switch/2
  Mux/1 -> Quadcopter model/2(init. cond.)
  (x,y,z,psi)/1 -> Manual Switch1/2

== system Consensus_Swarm/FOLLOWER 5/Agent Model ==
  (x,y,z,psi) : Inport
  Constant2 : Constant  Value=[0;-0;-40]  VectorParams1D=off
  Degrees to Radians : simulink_extras/Transformations/Degrees to Radians
  Demux1 : Demux  Outputs=6
  Flight Control System : Subsystem
      settings: PortSchema="{\"entries\":[{\"content\":{\"sides\":[{\"content\":{\"connectorIds\":[\"In1\",\"In2\"]},\"type\":\"ConnectorPlacement.EquallySpacedRectSide\",\"uuid\":\"8ffec179-99fb-4b4c-a09d-a73fa0154dea\"},{\"content\":{\"connectorIds\":[\"Out1\"],\"side\":\"RIGHT\"},\"type\":\"ConnectorPlacement.EquallySpacedRectSide\",\"uuid\":\"b9ff487d-1da1-449a-81c9-f1838b0d3727\"},{\"content\":{\"connectorIds\":[\"In3\"],\"side\":\"TOP\"},\"type\":\"ConnectorPlacement.EquallySpacedRectSide\",\"uuid\":\"1948ac9a-8b1f-4a62-833b-18e2b106d39d\"}]},\"type\":\"ConnectorPlacement.EquallySpacedConnector\",\"uuid\":\"fea635f7-9753-4696-bad7-e2485c1b5acc\"}],\"packageUris\":[\"http://schema.mathworks.com/mf0/Connector/R2020b\"],\"version\":\"1.0\"}"
  Manual Switch : ManualSwitch  CurrentSetting=0
  Manual Switch1 : ManualSwitch  CurrentSetting=0
  Mux : Mux  Inputs=2
  OL inputs : Constant  Value=[0;0;0;0]  VectorParams1D=off
  Position refs (x,y,z,psi) : Constant  Value=[20;20;-17;-45]  VectorParams1D=off
  Quadcopter model : Subsystem
      settings: PortSchema="{\"entries\":[{\"content\":{\"sides\":[{\"content\":{\"connectorIds\":[\"In1\"]},\"type\":\"ConnectorPlacement.EquallySpacedRectSide\",\"uuid\":\"c5c2dfb8-9ff8-4aa4-96a6-7fa0d886c51f\"},{\"content\":{\"connectorIds\":[\"Out1\"],\"side\":\"RIGHT\"},\"type\":\"ConnectorPlacement.EquallySpacedRectSide\",\"uuid\":\"2d7c7d5c-4ac5-4ebd-b09f-6a78733e851d\"},{\"content\":{\"connectorIds\":[\"In2\"],\"side\":\"TOP\"},\"type\":\"ConnectorPlacement.EquallySpacedRectSide\",\"uuid\":\"cf3a786d-06ed-46d4-985b-5c210afb13ec\"}]},\"type\":\"ConnectorPlacement.EquallySpacedConnector\",\"uuid\":\"cd57f0e6-7b9c-4392-8478-6e8af8e2560e\"}],\"packageUris\":[\"http://schema.mathworks.com/mf0/Connector/R2020b\"],\"version\":\"1.0\"}"
  Radians to Degrees : simulink_extras/Transformations/Radians to Degrees
  Radians to Degrees1 : simulink_extras/Transformations/Radians to Degrees
  Radians to Degrees2 : simulink_extras/Transformations/Radians to Degrees
  gamepad : Subsystem  Commented=on
  p(0) : Constant  Value=[90;90;-50]  VectorParams1D=off
  phi(t) : Scope
  psi(t) : Scope
  theta(t) : Scope
  x(t) : Scope
  y(t) : Scope
  z(t) : Scope
  Eta : Outport
  wires:
  Radians to Degrees2/1 -> psi(t)/1
  Quadcopter model/1(eta) -> Eta/1, Demux1/1, Flight Control System/2(eta)
  OL inputs/1 -> Manual Switch/1
  Demux1/2 -> y(t)/1
  Constant2/1 -> Degrees to Radians/1
  gamepad/1(gamepad input) -> Flight Control System/3(gamepad input)
  p(0)/1 -> Mux/1
  Degrees to Radians/1 -> Mux/2
  Demux1/1 -> x(t)/1
  Radians to Degrees/1 -> phi(t)/1
  Demux1/4 -> Radians to Degrees/1
  Manual Switch1/1 -> Flight Control System/1(Pos. refs)
  Radians to Degrees1/1 -> theta(t)/1
  Demux1/3 -> z(t)/1
  Demux1/6 -> Radians to Degrees2/1
  Manual Switch/1 -> Quadcopter model/1(Fz,mx,my,mz)
  Demux1/5 -> Radians to Degrees1/1
  Position refs (x,y,z,psi)/1 -> Manual Switch1/1
  Flight Control System/1(Fz,mx,my,mz) -> Manual Switch/2
  Mux/1 -> Quadcopter model/2(init. cond.)
  (x,y,z,psi)/1 -> Manual Switch1/2

== system Consensus_Swarm/Formatting/Axes to VR Axes ==
  Xe : Inport
  Demux : Demux  Outputs=3
      settings: DisplayOption=none
  Mux : Mux  Inputs=3
  rad-->deg1 : Gain  Gain=-1  SaturateOnIntegerOverflow=on  OutDataTypeStr=Inherit: Same as input  ParamDataTypeStr=Inherit: Same as input
  Xe VR : Outport  VectorParamsAs1DForOutWhenUnconnected=off
  wires:
  Xe/1 -> Demux/1
  Demux/1 -> Mux/1
  Demux/3 -> rad-->deg1/1
  Mux/1 -> Xe VR/1
  rad-->deg1/1 -> Mux/2
  Demux/2 -> Mux/3

== system Consensus_Swarm/Formatting/Axes to VR Axes Camera Chase ==
  Xe : Inport
  Demux : Demux  Outputs=3
      settings: DisplayOption=none
  Mux : Mux  Inputs=3
  rad-->deg1 : Gain  Gain=-1  SaturateOnIntegerOverflow=on  OutDataTypeStr=Inherit: Same as input  ParamDataTypeStr=Inherit: Same as input
  Xe VR : Outport  VectorParamsAs1DForOutWhenUnconnected=off
  wires:
  Xe/1 -> Demux/1
  Demux/1 -> Mux/1
  Demux/3 -> rad-->deg1/1
  Mux/1 -> Xe VR/1
  rad-->deg1/1 -> Mux/2
  Demux/2 -> Mux/3

== system Consensus_Swarm/Formatting/Axes to VR Axes Camera Iso ==
  Xe : Inport
  Demux : Demux  Outputs=3
      settings: DisplayOption=none
  Mux : Mux  Inputs=3
  rad-->deg1 : Gain  Gain=-1  SaturateOnIntegerOverflow=on  OutDataTypeStr=Inherit: Same as input  ParamDataTypeStr=Inherit: Same as input
  Xe VR : Outport  VectorParamsAs1DForOutWhenUnconnected=off
  wires:
  Demux/2 -> Mux/3
  rad-->deg1/1 -> Mux/2
  Mux/1 -> Xe VR/1
  Demux/3 -> rad-->deg1/1
  Demux/1 -> Mux/1
  Xe/1 -> Demux/1

== system Consensus_Swarm/Formatting/Axes to VR Axes1 ==
  Xe : Inport
  Demux : Demux  Outputs=3
      settings: DisplayOption=none
  Mux : Mux  Inputs=3
  rad-->deg1 : Gain  Gain=-1  SaturateOnIntegerOverflow=on  OutDataTypeStr=Inherit: Same as input  ParamDataTypeStr=Inherit: Same as input
  Xe VR : Outport  VectorParamsAs1DForOutWhenUnconnected=off
  wires:
  Xe/1 -> Demux/1
  Demux/1 -> Mux/1
  Demux/3 -> rad-->deg1/1
  Mux/1 -> Xe VR/1
  rad-->deg1/1 -> Mux/2
  Demux/2 -> Mux/3

== system Consensus_Swarm/Formatting/Axes to VR Axes2 ==
  Xe : Inport
  Demux : Demux  Outputs=3
      settings: DisplayOption=none
  Mux : Mux  Inputs=3
  rad-->deg1 : Gain  Gain=-1  SaturateOnIntegerOverflow=on  OutDataTypeStr=Inherit: Same as input  ParamDataTypeStr=Inherit: Same as input
  Xe VR : Outport  VectorParamsAs1DForOutWhenUnconnected=off
  wires:
  Xe/1 -> Demux/1
  Demux/1 -> Mux/1
  Demux/3 -> rad-->deg1/1
  Mux/1 -> Xe VR/1
  rad-->deg1/1 -> Mux/2
  Demux/2 -> Mux/3

== system Consensus_Swarm/Formatting/Axes to VR Axes3 ==
  Xe : Inport
  Demux : Demux  Outputs=3
      settings: DisplayOption=none
  Mux : Mux  Inputs=3
  rad-->deg1 : Gain  Gain=-1  SaturateOnIntegerOverflow=on  OutDataTypeStr=Inherit: Same as input  ParamDataTypeStr=Inherit: Same as input
  Xe VR : Outport  VectorParamsAs1DForOutWhenUnconnected=off
  wires:
  Xe/1 -> Demux/1
  Demux/1 -> Mux/1
  Demux/3 -> rad-->deg1/1
  Mux/1 -> Xe VR/1
  rad-->deg1/1 -> Mux/2
  Demux/2 -> Mux/3

== system Consensus_Swarm/Formatting/Axes to VR Axes4 ==
  Xe : Inport
  Demux : Demux  Outputs=3
      settings: DisplayOption=none
  Mux : Mux  Inputs=3
  rad-->deg1 : Gain  Gain=-1  SaturateOnIntegerOverflow=on  OutDataTypeStr=Inherit: Same as input  ParamDataTypeStr=Inherit: Same as input
  Xe VR : Outport  VectorParamsAs1DForOutWhenUnconnected=off
  wires:
  Xe/1 -> Demux/1
  Demux/1 -> Mux/1
  Demux/3 -> rad-->deg1/1
  Mux/1 -> Xe VR/1
  rad-->deg1/1 -> Mux/2
  Demux/2 -> Mux/3

== system Consensus_Swarm/Formatting/Axes to VR Axes5 ==
  Xe : Inport
  Demux : Demux  Outputs=3
      settings: DisplayOption=none
  Mux : Mux  Inputs=3
  rad-->deg1 : Gain  Gain=-1  SaturateOnIntegerOverflow=on  OutDataTypeStr=Inherit: Same as input  ParamDataTypeStr=Inherit: Same as input
  Xe VR : Outport  VectorParamsAs1DForOutWhenUnconnected=off
  wires:
  Xe/1 -> Demux/1
  Demux/1 -> Mux/1
  Demux/3 -> rad-->deg1/1
  Mux/1 -> Xe VR/1
  rad-->deg1/1 -> Mux/2
  Demux/2 -> Mux/3

== system Consensus_Swarm/Formatting/Euler to VR ==
  Euler Angles : Inport
  Axis Angle Vector : Subsystem
  Mux : Mux  Inputs=2
  Mux1 : Mux  Inputs=2
  Mux2 : Mux  Inputs=2
  Quaternion Multiplication (Pitch & Yaw) : aerolibutil/Quaternion Multiplication
  Quaternion Multiplication (Roll) : aerolibutil/Quaternion Multiplication
  Quaternion Normalization : Subsystem
  Quaternion Normalization1 : Subsystem
  Quaternion Normalization2 : Subsystem
  Selector : Selector  InputPortWidth=3  IndexOptions=Index vector (dialog)  Indices=[3]  OutputSizes=1
  Selector1 : Selector  InputPortWidth=3  IndexOptions=Index vector (dialog)  Indices=[2]  OutputSizes=1
  Selector2 : Selector  InputPortWidth=3  IndexOptions=Index vector (dialog)  Indices=[1]  OutputSizes=1
  Vr Pitch Axes : Constant  Value=[0 0 1]
  Vr Roll Axes : Constant  Value=[1 0 0]
  Vr Yaw Axes : Constant  Value=[0 -1 0]
  Axis Angle : Outport  VectorParamsAs1DForOutWhenUnconnected=off
  wires:
  Quaternion Multiplication (Roll)/1 -> Axis Angle Vector/1(e0)
  Axis Angle Vector/1(e0_norm) -> Axis Angle/1
  Quaternion Normalization/1(e0_norm) -> Quaternion Multiplication (Roll)/2
  Quaternion Normalization2/1(e0_norm) -> Quaternion Multiplication (Pitch & Yaw)/1
  Quaternion Normalization1/1(e0_norm) -> Quaternion Multiplication (Pitch & Yaw)/2
  Mux2/1 -> Quaternion Normalization2/1(e0)
  Mux1/1 -> Quaternion Normalization1/1(e0)
  Mux/1 -> Quaternion Normalization/1(e0)
  Selector/1 -> Mux2/1
  Vr Yaw Axes/1 -> Mux2/2
  Selector1/1 -> Mux1/1
  Vr Pitch Axes/1 -> Mux1/2
  Selector2/1 -> Mux/1
  Vr Roll Axes/1 -> Mux/2
  Euler Angles/1 -> Selector2/1, Selector1/1, Selector/1
  Quaternion Multiplication (Pitch & Yaw)/1 -> Quaternion Multiplication (Roll)/1

== system Consensus_Swarm/Formatting/Euler to VR1 ==
  Euler Angles : Inport
  Axis Angle Vector : Subsystem
  Mux : Mux  Inputs=2
  Mux1 : Mux  Inputs=2
  Mux2 : Mux  Inputs=2
  Quaternion Multiplication (Pitch & Yaw) : aerolibutil/Quaternion Multiplication
  Quaternion Multiplication (Roll) : aerolibutil/Quaternion Multiplication
  Quaternion Normalization : Subsystem
  Quaternion Normalization1 : Subsystem
  Quaternion Normalization2 : Subsystem
  Selector : Selector  InputPortWidth=3  IndexOptions=Index vector (dialog)  Indices=[3]  OutputSizes=1
  Selector1 : Selector  InputPortWidth=3  IndexOptions=Index vector (dialog)  Indices=[2]  OutputSizes=1
  Selector2 : Selector  InputPortWidth=3  IndexOptions=Index vector (dialog)  Indices=[1]  OutputSizes=1
  Vr Pitch Axes : Constant  Value=[0 0 1]
  Vr Roll Axes : Constant  Value=[1 0 0]
  Vr Yaw Axes : Constant  Value=[0 -1 0]
  Axis Angle : Outport  VectorParamsAs1DForOutWhenUnconnected=off
  wires:
  Quaternion Multiplication (Roll)/1 -> Axis Angle Vector/1(e0)
  Axis Angle Vector/1(e0_norm) -> Axis Angle/1
  Quaternion Normalization/1(e0_norm) -> Quaternion Multiplication (Roll)/2
  Quaternion Normalization2/1(e0_norm) -> Quaternion Multiplication (Pitch & Yaw)/1
  Quaternion Normalization1/1(e0_norm) -> Quaternion Multiplication (Pitch & Yaw)/2
  Mux2/1 -> Quaternion Normalization2/1(e0)
  Mux1/1 -> Quaternion Normalization1/1(e0)
  Mux/1 -> Quaternion Normalization/1(e0)
  Selector/1 -> Mux2/1
  Vr Yaw Axes/1 -> Mux2/2
  Selector1/1 -> Mux1/1
  Vr Pitch Axes/1 -> Mux1/2
  Selector2/1 -> Mux/1
  Vr Roll Axes/1 -> Mux/2
  Euler Angles/1 -> Selector2/1, Selector1/1, Selector/1
  Quaternion Multiplication (Pitch & Yaw)/1 -> Quaternion Multiplication (Roll)/1

== system Consensus_Swarm/Formatting/Euler to VR2 ==
  Euler Angles : Inport
  Axis Angle Vector : Subsystem
  Mux : Mux  Inputs=2
  Mux1 : Mux  Inputs=2
  Mux2 : Mux  Inputs=2
  Quaternion Multiplication (Pitch & Yaw) : aerolibutil/Quaternion Multiplication
  Quaternion Multiplication (Roll) : aerolibutil/Quaternion Multiplication
  Quaternion Normalization : Subsystem
  Quaternion Normalization1 : Subsystem
  Quaternion Normalization2 : Subsystem
  Selector : Selector  InputPortWidth=3  IndexOptions=Index vector (dialog)  Indices=[3]  OutputSizes=1
  Selector1 : Selector  InputPortWidth=3  IndexOptions=Index vector (dialog)  Indices=[2]  OutputSizes=1
  Selector2 : Selector  InputPortWidth=3  IndexOptions=Index vector (dialog)  Indices=[1]  OutputSizes=1
  Vr Pitch Axes : Constant  Value=[0 0 1]
  Vr Roll Axes : Constant  Value=[1 0 0]
  Vr Yaw Axes : Constant  Value=[0 -1 0]
  Axis Angle : Outport  VectorParamsAs1DForOutWhenUnconnected=off
  wires:
  Quaternion Multiplication (Roll)/1 -> Axis Angle Vector/1(e0)
  Axis Angle Vector/1(e0_norm) -> Axis Angle/1
  Quaternion Normalization/1(e0_norm) -> Quaternion Multiplication (Roll)/2
  Quaternion Normalization2/1(e0_norm) -> Quaternion Multiplication (Pitch & Yaw)/1
  Quaternion Normalization1/1(e0_norm) -> Quaternion Multiplication (Pitch & Yaw)/2
  Mux2/1 -> Quaternion Normalization2/1(e0)
  Mux1/1 -> Quaternion Normalization1/1(e0)
  Mux/1 -> Quaternion Normalization/1(e0)
  Selector/1 -> Mux2/1
  Vr Yaw Axes/1 -> Mux2/2
  Selector1/1 -> Mux1/1
  Vr Pitch Axes/1 -> Mux1/2
  Selector2/1 -> Mux/1
  Vr Roll Axes/1 -> Mux/2
  Euler Angles/1 -> Selector2/1, Selector1/1, Selector/1
  Quaternion Multiplication (Pitch & Yaw)/1 -> Quaternion Multiplication (Roll)/1

== system Consensus_Swarm/Formatting/Euler to VR3 ==
  Euler Angles : Inport
  Axis Angle Vector : Subsystem
  Mux : Mux  Inputs=2
  Mux1 : Mux  Inputs=2
  Mux2 : Mux  Inputs=2
  Quaternion Multiplication (Pitch & Yaw) : aerolibutil/Quaternion Multiplication
  Quaternion Multiplication (Roll) : aerolibutil/Quaternion Multiplication
  Quaternion Normalization : Subsystem
  Quaternion Normalization1 : Subsystem
  Quaternion Normalization2 : Subsystem
  Selector : Selector  InputPortWidth=3  IndexOptions=Index vector (dialog)  Indices=[3]  OutputSizes=1
  Selector1 : Selector  InputPortWidth=3  IndexOptions=Index vector (dialog)  Indices=[2]  OutputSizes=1
  Selector2 : Selector  InputPortWidth=3  IndexOptions=Index vector (dialog)  Indices=[1]  OutputSizes=1
  Vr Pitch Axes : Constant  Value=[0 0 1]
  Vr Roll Axes : Constant  Value=[1 0 0]
  Vr Yaw Axes : Constant  Value=[0 -1 0]
  Axis Angle : Outport  VectorParamsAs1DForOutWhenUnconnected=off
  wires:
  Quaternion Multiplication (Roll)/1 -> Axis Angle Vector/1(e0)
  Axis Angle Vector/1(e0_norm) -> Axis Angle/1
  Quaternion Normalization/1(e0_norm) -> Quaternion Multiplication (Roll)/2
  Quaternion Normalization2/1(e0_norm) -> Quaternion Multiplication (Pitch & Yaw)/1
  Quaternion Normalization1/1(e0_norm) -> Quaternion Multiplication (Pitch & Yaw)/2
  Mux2/1 -> Quaternion Normalization2/1(e0)
  Mux1/1 -> Quaternion Normalization1/1(e0)
  Mux/1 -> Quaternion Normalization/1(e0)
  Selector/1 -> Mux2/1
  Vr Yaw Axes/1 -> Mux2/2
  Selector1/1 -> Mux1/1
  Vr Pitch Axes/1 -> Mux1/2
  Selector2/1 -> Mux/1
  Vr Roll Axes/1 -> Mux/2
  Euler Angles/1 -> Selector2/1, Selector1/1, Selector/1
  Quaternion Multiplication (Pitch & Yaw)/1 -> Quaternion Multiplication (Roll)/1

== system Consensus_Swarm/Formatting/Euler to VR4 ==
  Euler Angles : Inport
  Axis Angle Vector : Subsystem
  Mux : Mux  Inputs=2
  Mux1 : Mux  Inputs=2
  Mux2 : Mux  Inputs=2
  Quaternion Multiplication (Pitch & Yaw) : aerolibutil/Quaternion Multiplication
  Quaternion Multiplication (Roll) : aerolibutil/Quaternion Multiplication
  Quaternion Normalization : Subsystem
  Quaternion Normalization1 : Subsystem
  Quaternion Normalization2 : Subsystem
  Selector : Selector  InputPortWidth=3  IndexOptions=Index vector (dialog)  Indices=[3]  OutputSizes=1
  Selector1 : Selector  InputPortWidth=3  IndexOptions=Index vector (dialog)  Indices=[2]  OutputSizes=1
  Selector2 : Selector  InputPortWidth=3  IndexOptions=Index vector (dialog)  Indices=[1]  OutputSizes=1
  Vr Pitch Axes : Constant  Value=[0 0 1]
  Vr Roll Axes : Constant  Value=[1 0 0]
  Vr Yaw Axes : Constant  Value=[0 -1 0]
  Axis Angle : Outport  VectorParamsAs1DForOutWhenUnconnected=off
  wires:
  Quaternion Multiplication (Roll)/1 -> Axis Angle Vector/1(e0)
  Axis Angle Vector/1(e0_norm) -> Axis Angle/1
  Quaternion Normalization/1(e0_norm) -> Quaternion Multiplication (Roll)/2
  Quaternion Normalization2/1(e0_norm) -> Quaternion Multiplication (Pitch & Yaw)/1
  Quaternion Normalization1/1(e0_norm) -> Quaternion Multiplication (Pitch & Yaw)/2
  Mux2/1 -> Quaternion Normalization2/1(e0)
  Mux1/1 -> Quaternion Normalization1/1(e0)
  Mux/1 -> Quaternion Normalization/1(e0)
  Selector/1 -> Mux2/1
  Vr Yaw Axes/1 -> Mux2/2
  Selector1/1 -> Mux1/1
  Vr Pitch Axes/1 -> Mux1/2
  Selector2/1 -> Mux/1
  Vr Roll Axes/1 -> Mux/2
  Euler Angles/1 -> Selector2/1, Selector1/1, Selector/1
  Quaternion Multiplication (Pitch & Yaw)/1 -> Quaternion Multiplication (Roll)/1
